simulink model "DCmotor_system_Explicit_MPC"  (R2024b)
settings: configuration reference "DCmotor_system_config" (kept outside this file)
undefined symbols (not defined in the file): controller_sw
settings Model: DataDictionary=sim_data_DCmotor_system.sldd  SILPILSystemUnderTest=refmodels  Creator=tshintai  LastModifiedBy=tshintai
settings ConfigSetRef: SourceName=DCmotor_system_config

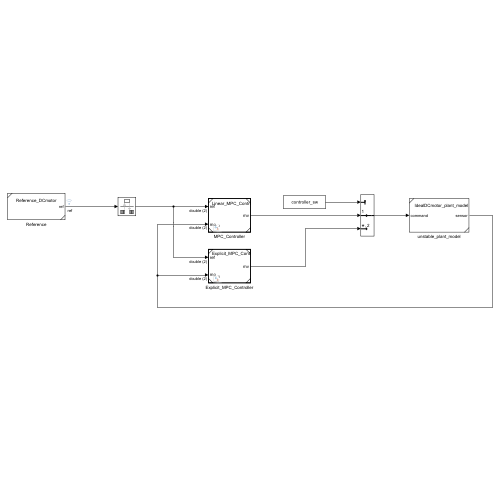
[thumbnail: Simulink's stored preview of the top-level diagram]
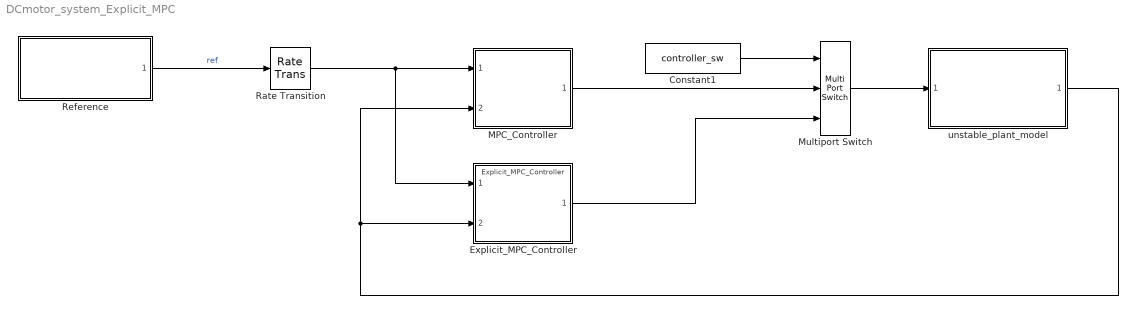
== system DCmotor_system_Explicit_MPC ==
  Constant1 : Constant  Value=controller_sw  OutDataTypeStr=uint32
  Explicit_MPC_Controller : ModelReference  ModelNameDialog=Explicit_MPC_Controller  SimulationMode=Normal  ModelReferenceVersion=8.0
  MPC_Controller : ModelReference  ModelNameDialog=Linear_MPC_Controller_for_DCmotor.slx  SimulationMode=Normal  ModelReferenceVersion=9.0
  Multiport Switch : MultiPortSwitch  Inputs=2  DiagnosticForDefault=None  SaturateOnIntegerOverflow=off  InputSameDT=off
  Rate Transition : RateTransition  OutPortSampleTime=TimeStep
  Reference : Subsystem  ReferencedSubsystem=Reference_DCmotor
  unstable_plant_model : Subsystem  ReferencedSubsystem=IdealDCmotor_plant_model
  wires:
  Rate Transition/1 -> MPC_Controller/1, Explicit_MPC_Controller/1
  unstable_plant_model/1 -> MPC_Controller/2, Explicit_MPC_Controller/2
  Constant1/1 -> Multiport Switch/1
  Reference/1 -> Rate Transition/1  "ref"
  MPC_Controller/1 -> Multiport Switch/2
  Multiport Switch/1 -> unstable_plant_model/1
  Explicit_MPC_Controller/1 -> Multiport Switch/3
